simulink model "thetaalpha"  (R2015b)
settings: Solver=ode1  StartTime=0.0  StopTime=50  FixedStep=0.002  RelTol=1e-3
InitFcn:
  | %% dynparams
  | Dr = 0.0015; %[Nms/rad]
  | Dp = 0.0005; %[Nms/rad]
  | 
  | mr = 0.095; %[kg] arm mass
  | mp = 0.024; %[kg] pendulum mass
  | Lr = 0.085; %[m]
  | Lp = 0.129; %[m]
  | 
  | Jr = mr*Lr^2/12;
  | Jp = (2.53+1.33)/2*1e-4;
  | 
  | Kt = 0.042; %[Nm/A]
  | Rm = 8.4; %[Ohm]
  | 
  | % Km = 0.042; %[Vs/rad] not used (back emf term), low speed means this is negligible.
  | 
  | 
  | Jt = Jr*Jp + mp*(Lp/2)^2*Jr + Jp*mp*Lr^2;
  | 
  | g = 9.81; %[m/s^2] gravity
undefined symbols (not defined in the file or in its folder): HIL
libraries: quarc_library x5
settings Model: SimulationMode=external  ExtModeTrigDuration=25001  Creator=felix  LastModifiedBy=SooJengTan
settings SolverCC: PositivePriorityOrder=on
settings DataIOCC: SaveFormat=Array
settings DebuggingCC: SolverPrmCheckMsg=warning
settings HardwareCC: ProdBitPerPointer=32  ProdLargestAtomicFloat=None  ProdIntDivRoundTo=Undefined  ProdEndianess=Unspecified  ProdWordSize=32  ProdHWDeviceType=32-bit Generic
settings RTWCC: SystemTargetFile=quarc_win64.tlc  TemplateMakefile=quarc_default_tmf  Description=QUARC Win64 Target
settings STFCustomTargetCC: CombineOutputUpdateFcns=on  CPPClassGenCompliant=off  GRTInterface=off
settings GRTTargetCC: ParMdlRefBuildCompliant=off  CompOptLevelCompliant=off  GeneratePreprocessorConditionals=Disable all  MatFileLogging=off  CPPClassGenCompliant=off  UseToolchainInfoCompliant=off  ExtMode=on  ExtModeMexFile=quarc_comm
settings ConfigComp: CovModelRefEnable=Off  CovSFcnEnable=off

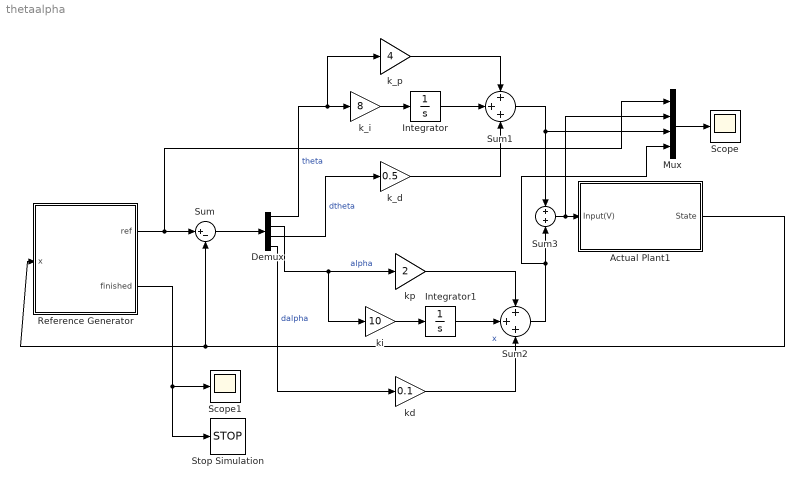
== system thetaalpha ==
  Actual Plant1 : Subsystem
  Demux : Demux
  Integrator : Integrator
  Integrator1 : Integrator
  Mux : Mux
  Reference Generator : MATLAB Function  TreatAsAtomicUnit=on
  Scope : Scope
  Scope1 : Scope
  Stop Simulation : Stop
  Sum : Sum  Inputs=|+-
  Sum1 : Sum  Inputs=+++
  Sum2 : Sum  Inputs=+++
  Sum3 : Sum  Inputs=+|+
  k_d : Gain  Gain=0.5
  k_i : Gain  Gain=8
  k_p : Gain  Gain=4
  kd : Gain  Gain=0.1
  ki : Gain  Gain=10
  kp : Gain  Gain=2
  wires:
  Actual Plant1/1(State) -> Sum/2, Reference Generator/1(x)  "x"
  Reference Generator/1(ref) -> Mux/1, Sum/1
  Reference Generator/2(finished) -> Stop Simulation/1, Scope1/1
  k_i/1 -> Integrator/1
  Demux/1 -> k_i/1, k_p/1  "theta"
  k_p/1 -> Sum1/1
  Integrator/1 -> Sum1/2
  Demux/3 -> k_d/1  "dtheta"
  k_d/1 -> Sum1/3
  Sum/1 -> Demux/1
  ki/1 -> Integrator1/1
  kp/1 -> Sum2/1
  Integrator1/1 -> Sum2/2
  kd/1 -> Sum2/3
  Demux/2 -> ki/1, kp/1  "alpha"
  Demux/4 -> kd/1  "dalpha"
  Sum3/1 -> Mux/2, Actual Plant1/1(Input(V))
  Sum1/1 -> Mux/3, Sum3/1
  Mux/1 -> Scope/1
  Sum2/1 -> Mux/4, Sum3/2

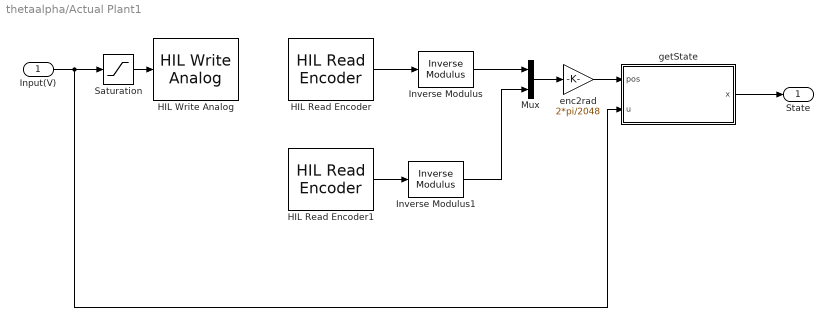
== system thetaalpha/Actual Plant1 ==
  Input(V) : Inport
  HIL Read Encoder : quarc_library/Data Acquisition/Generic/Immediate I//O/HIL Read Encoder  object_name=HIL-1  channels=0  sample_time=qc_get_step_size  active=on  vector_output=off  data_type_mode=Inherit via back propagation  data_type=double
  HIL Read Encoder1 : quarc_library/Data Acquisition/Generic/Immediate I//O/HIL Read Encoder  object_name=HIL-1  channels=1  sample_time=qc_get_step_size  active=on  vector_output=off  data_type_mode=Inherit via back propagation  data_type=double
  HIL Write Analog : quarc_library/Data Acquisition/Generic/Immediate I//O/HIL Write Analog  object_name=HIL-1  channels=0  sample_time=-1  active=off  vector_input=off
  Inverse Modulus : quarc_library/Discontinuities/Inverse Modulus  modulus=65535  output_derivative=off  output_revolutions=off  max_x=Inf  min_x=-Inf
  Inverse Modulus1 : quarc_library/Discontinuities/Inverse Modulus  modulus=65535  output_derivative=off  output_revolutions=off  max_x=Inf  min_x=-Inf
  Mux : Mux  Inputs=2
  Saturation : Saturate  UpperLimit=5  LowerLimit=-5
  enc2rad : Gain  Gain=2*pi/2048
  getState : Subsystem
  State : Outport
  wires:
  HIL Read Encoder/1 -> Inverse Modulus/1
  Inverse Modulus/1 -> Mux/1
  HIL Read Encoder1/1 -> Inverse Modulus1/1
  Inverse Modulus1/1 -> Mux/2
  Mux/1 -> enc2rad/1
  Saturation/1 -> HIL Write Analog/1
  enc2rad/1 -> getState/1(pos)
  getState/1(x) -> State/1
  Input(V)/1 -> Saturation/1, getState/2(u)

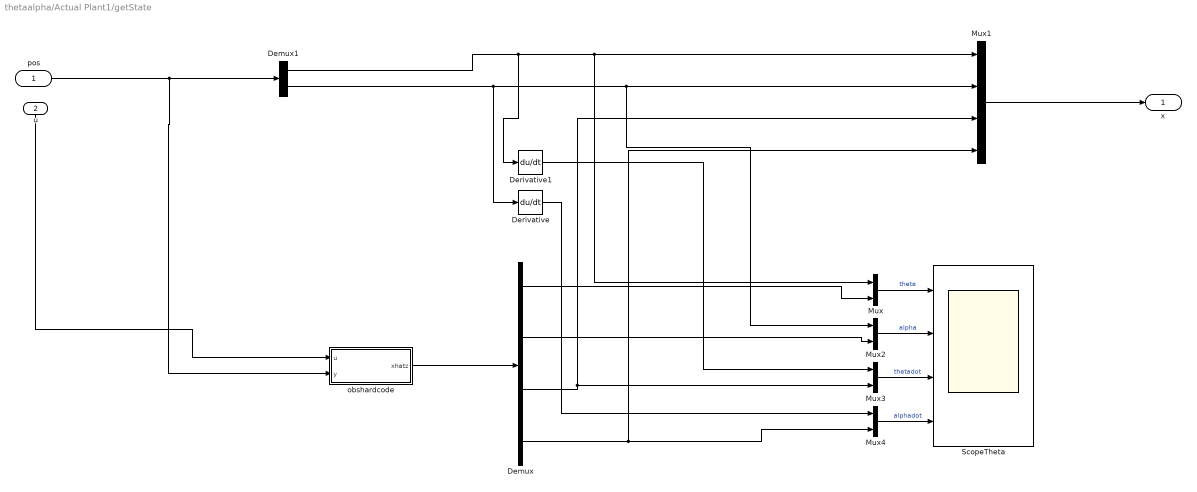
== system thetaalpha/Actual Plant1/getState ==
  pos : Inport
  u : Inport  Port=2
  Demux : Demux
  Demux1 : Demux  Outputs=2
  Derivative : Derivative
  Derivative1 : Derivative
  Mux{,2..4} (4 alike) : Mux  Inputs=2
  Mux1 : Mux
  ScopeTheta : Scope  NumInputPorts=4
  obshardcode : Subsystem
  x : Outport
  wires:
  Mux1/1 -> x/1
  pos/1 -> obshardcode/2(y), Demux1/1
  u/1 -> obshardcode/1(u)
  Mux/1 -> ScopeTheta/1  "theta"
  Mux4/1 -> ScopeTheta/4  "alphadot"
  Mux3/1 -> ScopeTheta/3  "thetadot"
  Mux2/1 -> ScopeTheta/2  "alpha"
  Demux/1 -> Mux/2
  Demux/4 -> Mux1/4, Mux4/2
  Demux/2 -> Mux2/2
  Demux/3 -> Mux3/2, Mux1/3
  Demux1/1 -> Derivative1/1, Mux1/1, Mux/1
  Derivative1/1 -> Mux3/1
  obshardcode/1(xhatz) -> Demux/1
  Demux1/2 -> Derivative/1, Mux2/1, Mux1/2
  Derivative/1 -> Mux4/1

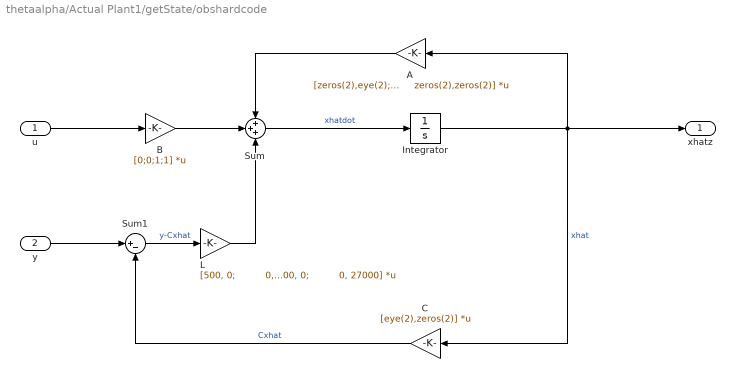
== system thetaalpha/Actual Plant1/getState/obshardcode ==
  u : Inport  PortDimensions=1
  y : Inport  Port=2  PortDimensions=2
  A : Gain  Gain=|  Multiplication=Matrix(K*u)
      | [zeros(2),eye(2);
      |       zeros(2),zeros(2)]
  B : Gain  Gain=[0;0;1;1]  Multiplication=Matrix(K*u)
  C : Gain  Gain=[eye(2),zeros(2)]  Multiplication=Matrix(K*u)
  Integrator : Integrator  InitialCondition=zeros(4,1)
  L : Gain  Gain=|  Multiplication=Matrix(K*u)
      | [500, 0;
      |          0, 500;
      |          27000, 0;
      |          0, 27000]
  Sum : Sum  Inputs=+++
  Sum1 : Sum  Inputs=|+-
  xhatz : Outport
  wires:
  L/1 -> Sum/3
  Sum1/1 -> L/1  "y-Cxhat"
  C/1 -> Sum1/2  "Cxhat"
  y/1 -> Sum1/1
  A/1 -> Sum/1
  Integrator/1 -> A/1, C/1, xhatz/1  "xhat"
  B/1 -> Sum/2
  Sum/1 -> Integrator/1  "xhatdot"
  u/1 -> B/1

== matlab function thetaalpha/Reference Generator ==
  data: x input size=4; ref output; finished output
function [ref, finished] = REFGEN(x)
%#codegen
%% Crane Reference Generator: For AMME3500 Lab 3 (2016)
% 
% Generates three `waypoints' for the crane's horizontal linkage. When the
% state is settled close to the reference at close to zero velocity, the
% next waypoint is given (the change is a step change). When all the waypoints 
% have been reached, then the task is finished.
%
% Let q1 be the horizontal linkage, and q2 be the vertical (unactuated)
% linkage on the pendulum.
%
%
% Input: 
% x         [4x1] [q1; q2; q1dot; q2dot] (rad and rad/s)
%
% Output:
% ref       [1x1] q1 reference position (rad)
%

%% Declare variables
% Persistent variables
persistent n 
persistent done
if(isempty(n))
    n = 1; % start at first waypoint
    done = false;
end

ref = zeros(4,1);

% Local variables
waypoints = [30; -60; 45; 0]*pi/180; % reference waypoints
posTol = 1*pi/180; % [rad] position tolerance
posTolPend = posTol;
velTol = 0.05; % [rad/s] velocity tolerance

%% Detect successful arrival at waypoint
if(~done) % only check for arrival if not done
    if(abs(waypoints(n)-x(1)) <= posTol) % q1 arrived
        if(abs(x(2)) <= posTolPend) % q2 pointing straight down
            if(abs(x(3)) <= velTol && abs(x(4)) <= velTol) % q1 and q2 stationary
                n = n + 1;
                if n > length(waypoints);
                    done = true;
                end
            end
        end
    end
end

%% Output reference
if(~done)
    ref(1) = waypoints(n);
    finished = done;
else
    ref(1) = waypoints(end);
    finished = done;
end
